simulink model "untitled1"  (R2020a)
settings: Solver=FixedStepDiscrete  StartTime=0.0  StopTime=10.0  FixedStep=0.1  RelTol=1e-3  EnableMultiTasking=on
settings Model: Creator=91968  LastModifiedBy=91968
settings SolverCC: AutoInsertRateTranBlk=on
settings DataIOCC: LimitDataPoints=on
settings OptimizationCC: LifeSpan=inf
settings DebuggingCC: AllowSymbolicDim=off  SFUnexpectedBacktrackingDiag=warning  SFNoUnconditionalDefaultTransitionDiag=warning  SFExecutionAtInitializationDiag=none  ArithmeticOperatorsInVariantConditions=warning
settings SFSimCC: SimUseLocalCustomCode=off  CustomCodeUndefinedFunction=UseInterfaceOnly
settings RTWCC: RTWUseLocalCustomCode=off
settings CodeAppCC: StateflowObjectComments=on
settings GRTTargetCC: TargetLangStandard=C89/C90 (ANSI)
settings ConfigComp: CovMetricSettings=dw  CovHtmlReporting=on  CovSaveCumulativeToWorkspaceVar=on  CovSaveSingleToWorkspaceVar=on  CovShowResultsExplorer=off  CovExternalEMLEnable=off  CovSFcnEnable=off

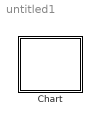
== system untitled1 ==
  Chart : Stateflow chart  TreatAsAtomicUnit=on

== stateflow chart untitled1/Chart ==
  state ACTUATOR_LOGIC
    state ACC_OFF
      send(ACC_OFF, ACC_LOGIC);
      throttle = driver_throttle;
      break_pdl = driver_break;
      mode =driverControl;
    state ACC_ON
      en: ss_button = false;
      en: send(ACC_ON, ACC_LOGIC);
      du: throttle = ACC_throttle;
      du: break_pdl = ACC_break;
      state SS_BUTTON_UNPRESSED
        en: ss_button = false;
      state SS_BUTTON_PRESSED
        en: ss_button = true;
        en: set_speed = input_Speed;
      (default) -> SS_BUTTON_UNPRESSED
      SS_BUTTON_UNPRESSED -> SS_BUTTON_PRESSED : [set_cc>0]
    (default) -> ACC_OFF
    ACC_OFF -> ACC_ON : [veh_speed>30]
    ACC_ON -> ACC_OFF : [driver_break>0]
  events: set_button local FUNCTION_CALL_EVENT
